simulink model "CPGnode"  (R2021b)
settings: Solver=VariableStepAuto  StartTime=0.0  StopTime=10.0  RelTol=1e-3
values from neighbouring files (symbols this model uses):
  ar = 2    [Snake5animal.m]    (also in animal.m; parameters.m)
  ax = 2    [Snake5animal.m]    (also in animal.m; parameters.m)
  omega = ones(1,N)*0.6*pi    [Snake5animal.m]    (also in animal.m = ones(3,3)*2; parameters.m = ones(3,3)*0.5)
  omegaM = ones(N,N)*2    [Snake5animal.m]
  phiM = ones(N,N)*PHI    [Snake5animal.m]
  R = [R1 R2 R3 R4 R5]    [Snake5animal.m]
  X = zeros(1,N)    [Snake5animal.m]
settings Model: Creator=xizh0002  LastModifiedBy=xizh0002

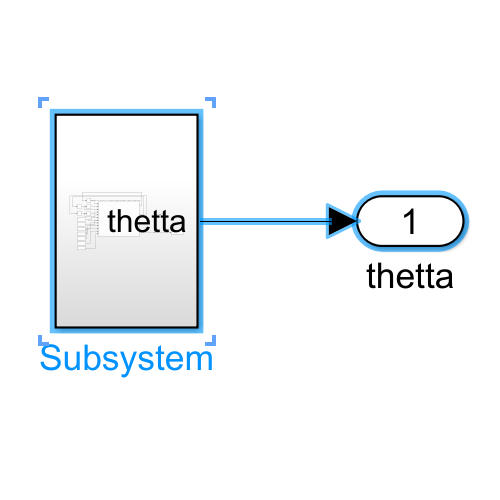
[thumbnail: Simulink's stored preview of the top-level diagram]
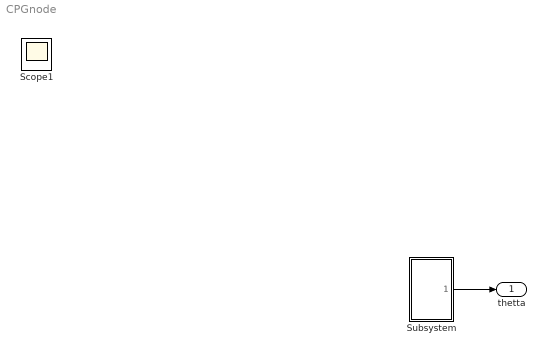
== system CPGnode ==
  Subsystem : Subsystem
  thetta : Outport
  Scope1 : Scope
  wires:
  Subsystem/1(thetta) -> thetta/1

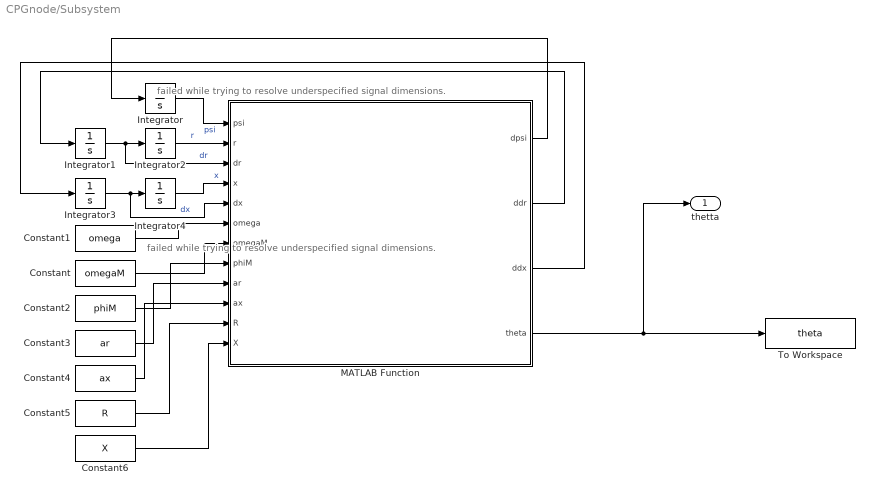
== system CPGnode/Subsystem ==
  note: failed while trying to resolve underspecified signal dimensions.
  note: failed while trying to resolve underspecified signal dimensions.
  Constant : Constant  Value=omegaM
  Constant1 : Constant  Value=omega
  Constant2 : Constant  Value=phiM
  Constant3 : Constant  Value=ar
  Constant4 : Constant  Value=ax
  Constant5 : Constant  Value=R
  Constant6 : Constant  Value=X
  Integrator{,1..4} (5 alike) : Integrator
  MATLAB Function : MATLAB Function  TreatAsAtomicUnit=on
  To Workspace : ToWorkspace  VariableName=theta  SaveFormat=Timeseries  SampleTime=-1
  thetta : Outport
  wires:
  Constant1/1 -> MATLAB Function/6(omega)
  Constant/1 -> MATLAB Function/7(omegaM)
  Integrator3/1 -> Integrator4/1, MATLAB Function/5(dx)  "dx"
  Integrator1/1 -> MATLAB Function/3(dr), Integrator2/1  "dr"
  Constant3/1 -> MATLAB Function/9(ar)
  MATLAB Function/2(ddr) -> Integrator1/1
  Integrator/1 -> MATLAB Function/1(psi)  "psi"
  MATLAB Function/1(dpsi) -> Integrator/1
  Integrator4/1 -> MATLAB Function/4(x)  "x"
  Constant5/1 -> MATLAB Function/11(R)
  MATLAB Function/3(ddx) -> Integrator3/1
  Constant4/1 -> MATLAB Function/10(ax)
  Integrator2/1 -> MATLAB Function/2(r)  "r"
  Constant2/1 -> MATLAB Function/8(phiM)
  Constant6/1 -> MATLAB Function/12(X)
  MATLAB Function/4(theta) -> thetta/1, To Workspace/1

== matlab function CPGnode/Subsystem/MATLAB Function ==
  data: psi input; dpsi output; r input; dr input; x input; dx input; omega input; omegaM input; phiM input; ar input; ax input; R input; X input; ddr output; ddx output; theta output
function [dpsi,ddr,ddx,theta] = oscillator(psi, r, dr, x, dx, omega, omegaM, phiM, ar, ax, R, X)
N = 5;
dpsi = zeros(1,N);
ddr = zeros(1,N);
ddx = zeros(1,N);
theta = zeros(1,N);
for i=1:N
    %dpsi
    for j=1:N
        dpsi(i) = omegaM(i,j)*r(j)*sin(psi(j)-psi(i)-phiM(i,j)); 
    end
    dpsi(i) = omega(i) + dpsi(i);
    ddr(i) = ar*(ar/4*(R(i)-r(i)-dr(i)));
    ddx(i) = ax*(ax/4*(X(i)-x(i)-dx(i)));
    theta(i) = x(i) + r(i)*cos(psi(i));
end
